simulink model "multilevelinverter1"  (R2014a)
settings: Solver=ode23tb  StartTime=0.0  StopTime=1  RelTol=1e-3
undefined symbols (not defined in the file): a, Gn, Ipvn, Iscn, k, Ki, Kv, Npp, Ns, Nss, q, Rp, Rs, Tn, Vocn
libraries: powerlib x102, simulink x34, dsparch4 x12, powerlib_extras x12, powerlib_meascontrol x3
(part 2 of 2)

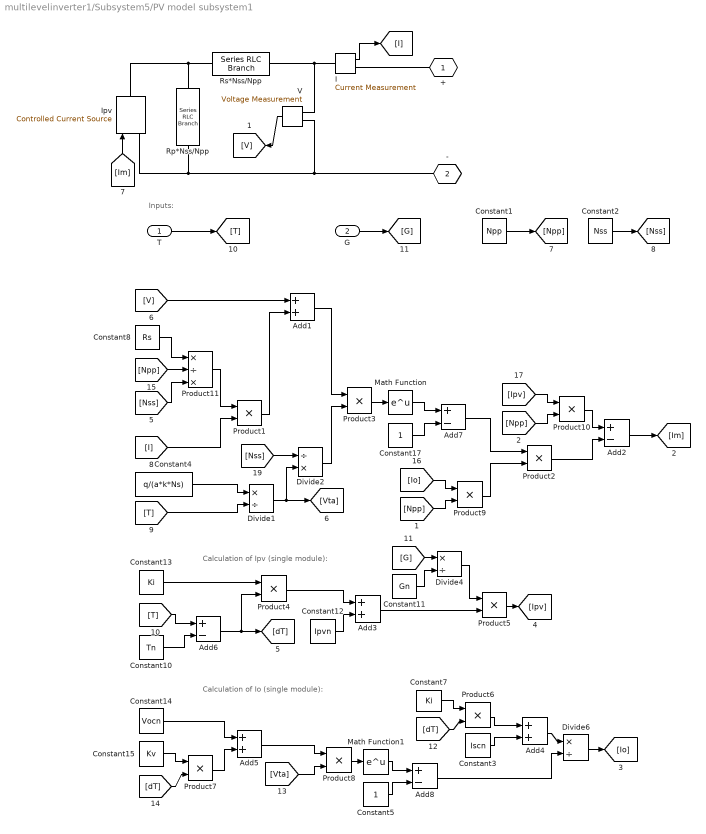
== system multilevelinverter1/Subsystem5/PV model subsystem1 ==
  note: Inputs:
  note: Calculation of Ipv (single module):
  note: Calculation of Io (single module):
  T : Inport
  G : Inport  Port=2
  Add{1,3..5} (4 alike) : Sum
  Add{2,6..8} (4 alike) : Sum  Inputs=+-
  Constant1 : Constant  Value=Npp
  Constant10 : Constant  Value=Tn
  Constant11 : Constant  Value=Gn
  Constant12 : Constant  Value=Ipvn
  Constant13 : Constant  Value=Ki
  Constant14 : Constant  Value=Vocn
  Constant15 : Constant  Value=Kv
  Constant17 : Constant
  Constant2 : Constant  Value=Nss
  Constant3 : Constant  Value=Iscn
  Constant4 : Constant  Value=q/(a*k*Ns)
  Constant5 : Constant
  Constant7 : Constant  Value=Ki
  Constant8 : Constant  Value=Rs
  Divide1 : Product  Inputs=*/
  Divide2 : Product  Inputs=/*
  Divide4 : Product  Inputs=*/
  Divide6 : Product  Inputs=*/
  I : powerlib/Measurements/Current Measurement  PhasorSimulation=off  OutputType=Complex  PSBequivalent=0
  Ipv : powerlib/Electrical Sources/Controlled Current Source  Initialize=on  Source_Type=DC  Amplitude=00  Phase=0  Frequency=0  Measurements=None
  Math Function : Math  SaturateOnIntegerOverflow=on
  Math Function1 : Math  SaturateOnIntegerOverflow=on
  Product{1..10} (10 alike) : Product  RndMeth=Zero
  Product11 : Product  Inputs=*/*  RndMeth=Zero
  Rp*Nss/Npp : powerlib/Elements/Series RLC Branch  LConnTagsString=__new0  RConnTagsString=__new0  BranchType=R  Resistance=Rp*Nss/Npp  Inductance=1e-3  SetiL0=off  InitialCurrent=0  Capacitance=1e-6  Setx0=off  InitialVoltage=0  Measurements=None
  Rs*Nss/Npp : powerlib/Elements/Series RLC Branch  LConnTagsString=__new0  RConnTagsString=__new0  BranchType=R  Resistance=Rs*Nss/Npp  Inductance=1e-3  SetiL0=off  InitialCurrent=0  Capacitance=1e-6  Setx0=off  InitialVoltage=0  Measurements=None
  "V " : powerlib/Measurements/Voltage Measurement  PhasorSimulation=off  OutputType=Complex  PSBequivalent=0
  + : PMIOPort  Port=1  Side=Right
  - : PMIOPort  Port=2  Side=Right
  wires:
  I/1 -> [I]
  "V "/1 -> [V]
  [Im] -> Ipv/1
  G/1 -> [G]
  T/1 -> [T]
  Constant10/1 -> Add6/2
  [T] -> Add6/1
  [I] -> Product1/2
  Constant4/1 -> Divide1/1
  [T] -> Divide1/2
  [V] -> Add1/1
  Product3/1 -> Math Function/1
  Add2/1 -> [Im]
  Add1/1 -> Product3/1
  [G] -> Divide4/1
  Constant11/1 -> Divide4/2
  Constant13/1 -> Product4/1
  [dT] -> Product6/2
  Constant7/1 -> Product6/1
  [dT] -> Product7/2
  Constant14/1 -> Add5/1
  Product8/1 -> Math Function1/1
  Add5/1 -> Product8/1
  Constant17/1 -> Add7/2
  Add7/1 -> Product2/1
  Constant5/1 -> Add8/2
  Math Function1/1 -> Add8/1
  Divide6/1 -> [Io]
  Product5/1 -> [Ipv]
  Product1/1 -> Add1/2
  Math Function/1 -> Add7/1
  Product4/1 -> Add3/1
  Add3/1 -> Product5/2
  Divide4/1 -> Product5/1
  Product7/1 -> Add5/2
  Constant15/1 -> Product7/1
  [Vta] -> Product8/2
  Add8/1 -> Divide6/2
  Constant3/1 -> Add4/2
  Product6/1 -> Add4/1
  Constant12/1 -> Add3/2
  Product2/1 -> Add2/2
  Product9/1 -> Product2/2
  [Io] -> Product9/1
  [Npp] -> Product9/2
  Constant1/1 -> [Npp]
  Constant2/1 -> [Nss]
  [Ipv] -> Product10/1
  [Npp] -> Product10/2
  Product10/1 -> Add2/1
  Constant8/1 -> Product11/1
  [Npp] -> Product11/2
  [Nss] -> Product11/3
  Product11/1 -> Product1/1
  [Nss] -> Divide2/1
  Divide1/1 -> Divide2/2, [Vta]
  Divide2/1 -> Product3/2
  Add6/1 -> [dT], Product4/2
  Add4/1 -> Divide6/1
  connections:
  I/LConn1 -- "V "/LConn1 -- Rs*Nss/Npp/RConn1
  -/RConn1 -- Rp*Nss/Npp/RConn1 -- Ipv/LConn1 -- "V "/LConn2
  Ipv/RConn1 -- Rs*Nss/Npp/LConn1 -- Rp*Nss/Npp/LConn1
  +/RConn1 -- I/RConn1

== system multilevelinverter1/Subsystem6/PV Boost Converter1 ==
  Analog Filter Design : dsparch4/Analog Filter Design  method=Butterworth  filttype=Lowpass  N=8  Wlo=30  Whi=80  Rp=2  Rs=40
  Analog Filter Design1 : dsparch4/Analog Filter Design  method=Butterworth  filttype=Lowpass  N=8  Wlo=30  Whi=80  Rp=2  Rs=40
  Current Measurement : powerlib/Measurements/Current Measurement  PhasorSimulation=off  OutputType=Complex  PSBequivalent=0
  Diode : powerlib/Power Electronics/Diode  Ron=0.001  Lon=0  Vf=0.8  IC=0  UseSnubber=off  Rs=500  Cs=250e-9  Measurements=on
  MPPT : Subsystem
  Mosfet : powerlib/Power Electronics/Mosfet  Ron=0.1  Lon=0  Rd=0.01  Vfd=0  IC=0  Rs=1e5  Cs=inf  Measurements=on
  PI CONTOLER : Subsystem
  Relational Operator1 : RelationalOperator  Operator=<=  OutDataTypeStr=boolean
  Repeating Sequence : simulink/Sources/Repeating Sequence  rep_seq_t=[0 0.0001 0.0002]  rep_seq_y=[0 10 0]
  Scope{1..3,8} (4 alike) : Scope
      Scope1 settings: SaveName=ScopeData2
      Scope2 settings: SaveName=ScopeData3
      Scope3 settings: YMin=-20  YMax=100  SaveName=ScopeData12
      Scope8 settings: YMin=47.1  YMax=48.9  SaveName=ScopeData4
  Series RLC Branch : powerlib/Elements/Series RLC Branch  LConnTagsString=__new0  RConnTagsString=__new0  BranchType=L  Resistance=1  Inductance=1e-3  SetiL0=off  InitialCurrent=0  Capacitance=1e-6  Setx0=off  InitialVoltage=0  Measurements=None
  Series RLC Branch1 : powerlib/Elements/Series RLC Branch  LConnTagsString=__new0  RConnTagsString=__new0  BranchType=C  Resistance=1  Inductance=12e-3  SetiL0=off  InitialCurrent=0  Capacitance=2200e-6  Setx0=off  InitialVoltage=0  Measurements=None
  Voltage Measurement1 : powerlib/Measurements/Voltage Measurement  PhasorSimulation=off  OutputType=Complex  PSBequivalent=0
  Voltage Measurement2 : powerlib/Measurements/Voltage Measurement  PhasorSimulation=off  OutputType=Complex  PSBequivalent=0
  + : PMIOPort  Port=1  Side=Right
  - : PMIOPort  Port=2  Side=Right
  Vpv+ : PMIOPort  Tag=PMCPort  Port=3  Side=Left
  Vpv- : PMIOPort  Tag=PMCPort  Port=4  Side=Left
  wires:
  Analog Filter Design1/1 -> MPPT/1(V)
  Analog Filter Design/1 -> MPPT/2(I)
  MPPT/1(D) -> Relational Operator1/2
  Relational Operator1/1 -> Scope1/1
  Repeating Sequence/1 -> Scope2/1, Relational Operator1/1
  Current Measurement/1 -> Analog Filter Design/1
  Voltage Measurement1/1 -> Scope8/1, [A1]
  [A1] -> PI CONTOLER/1(In1)
  PI CONTOLER/1(Out1) -> [G]
  Voltage Measurement2/1 -> Scope3/1, Analog Filter Design1/1
  [G] -> Mosfet/1
  connections:
  Current Measurement/LConn1 -- Vpv+/RConn1
  Diode/RConn1 -- Voltage Measurement1/LConn1 -- +/RConn1 -- Series RLC Branch1/LConn1
  Series RLC Branch/LConn1 -- Current Measurement/RConn1 -- Voltage Measurement2/LConn1
  Series RLC Branch1/RConn1 -- Voltage Measurement1/LConn2 -- -/RConn1 -- Mosfet/RConn1 -- Voltage Measurement2/LConn2 -- Vpv-/RConn1
  Diode/LConn1 -- Mosfet/LConn1 -- Series RLC Branch/RConn1

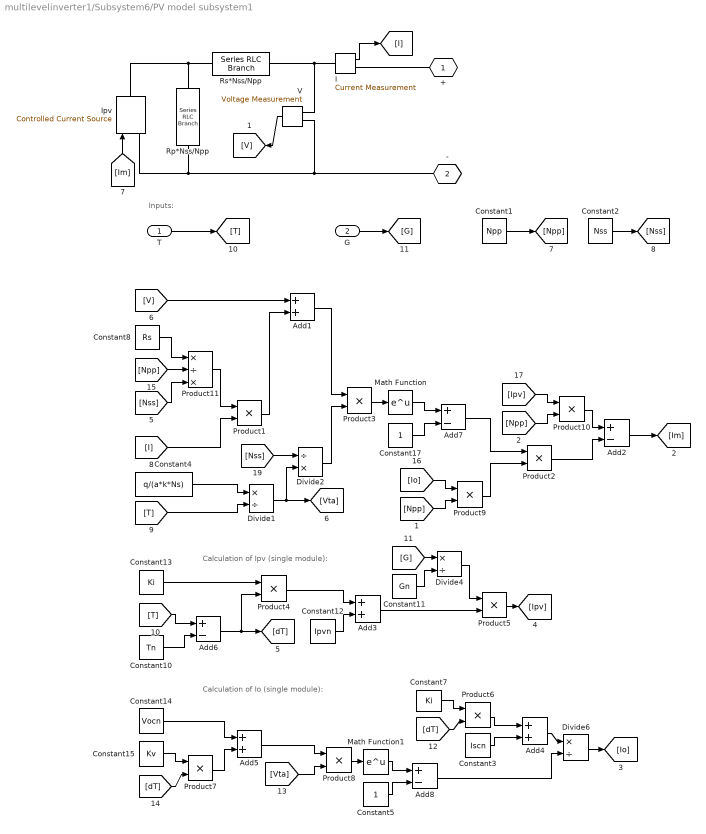
== system multilevelinverter1/Subsystem6/PV model subsystem1 ==
  note: Inputs:
  note: Calculation of Ipv (single module):
  note: Calculation of Io (single module):
  T : Inport
  G : Inport  Port=2
  Add{1,3..5} (4 alike) : Sum
  Add{2,6..8} (4 alike) : Sum  Inputs=+-
  Constant1 : Constant  Value=Npp
  Constant10 : Constant  Value=Tn
  Constant11 : Constant  Value=Gn
  Constant12 : Constant  Value=Ipvn
  Constant13 : Constant  Value=Ki
  Constant14 : Constant  Value=Vocn
  Constant15 : Constant  Value=Kv
  Constant17 : Constant
  Constant2 : Constant  Value=Nss
  Constant3 : Constant  Value=Iscn
  Constant4 : Constant  Value=q/(a*k*Ns)
  Constant5 : Constant
  Constant7 : Constant  Value=Ki
  Constant8 : Constant  Value=Rs
  Divide1 : Product  Inputs=*/
  Divide2 : Product  Inputs=/*
  Divide4 : Product  Inputs=*/
  Divide6 : Product  Inputs=*/
  I : powerlib/Measurements/Current Measurement  PhasorSimulation=off  OutputType=Complex  PSBequivalent=0
  Ipv : powerlib/Electrical Sources/Controlled Current Source  Initialize=on  Source_Type=DC  Amplitude=00  Phase=0  Frequency=0  Measurements=None
  Math Function : Math  SaturateOnIntegerOverflow=on
  Math Function1 : Math  SaturateOnIntegerOverflow=on
  Product{1..10} (10 alike) : Product  RndMeth=Zero
  Product11 : Product  Inputs=*/*  RndMeth=Zero
  Rp*Nss/Npp : powerlib/Elements/Series RLC Branch  LConnTagsString=__new0  RConnTagsString=__new0  BranchType=R  Resistance=Rp*Nss/Npp  Inductance=1e-3  SetiL0=off  InitialCurrent=0  Capacitance=1e-6  Setx0=off  InitialVoltage=0  Measurements=None
  Rs*Nss/Npp : powerlib/Elements/Series RLC Branch  LConnTagsString=__new0  RConnTagsString=__new0  BranchType=R  Resistance=Rs*Nss/Npp  Inductance=1e-3  SetiL0=off  InitialCurrent=0  Capacitance=1e-6  Setx0=off  InitialVoltage=0  Measurements=None
  "V " : powerlib/Measurements/Voltage Measurement  PhasorSimulation=off  OutputType=Complex  PSBequivalent=0
  + : PMIOPort  Port=1  Side=Right
  - : PMIOPort  Port=2  Side=Right
  wires:
  I/1 -> [I]
  "V "/1 -> [V]
  [Im] -> Ipv/1
  G/1 -> [G]
  T/1 -> [T]
  Constant10/1 -> Add6/2
  [T] -> Add6/1
  [I] -> Product1/2
  Constant4/1 -> Divide1/1
  [T] -> Divide1/2
  [V] -> Add1/1
  Product3/1 -> Math Function/1
  Add2/1 -> [Im]
  Add1/1 -> Product3/1
  [G] -> Divide4/1
  Constant11/1 -> Divide4/2
  Constant13/1 -> Product4/1
  [dT] -> Product6/2
  Constant7/1 -> Product6/1
  [dT] -> Product7/2
  Constant14/1 -> Add5/1
  Product8/1 -> Math Function1/1
  Add5/1 -> Product8/1
  Constant17/1 -> Add7/2
  Add7/1 -> Product2/1
  Constant5/1 -> Add8/2
  Math Function1/1 -> Add8/1
  Divide6/1 -> [Io]
  Product5/1 -> [Ipv]
  Product1/1 -> Add1/2
  Math Function/1 -> Add7/1
  Product4/1 -> Add3/1
  Add3/1 -> Product5/2
  Divide4/1 -> Product5/1
  Product7/1 -> Add5/2
  Constant15/1 -> Product7/1
  [Vta] -> Product8/2
  Add8/1 -> Divide6/2
  Constant3/1 -> Add4/2
  Product6/1 -> Add4/1
  Constant12/1 -> Add3/2
  Product2/1 -> Add2/2
  Product9/1 -> Product2/2
  [Io] -> Product9/1
  [Npp] -> Product9/2
  Constant1/1 -> [Npp]
  Constant2/1 -> [Nss]
  [Ipv] -> Product10/1
  [Npp] -> Product10/2
  Product10/1 -> Add2/1
  Constant8/1 -> Product11/1
  [Npp] -> Product11/2
  [Nss] -> Product11/3
  Product11/1 -> Product1/1
  [Nss] -> Divide2/1
  Divide1/1 -> Divide2/2, [Vta]
  Divide2/1 -> Product3/2
  Add6/1 -> [dT], Product4/2
  Add4/1 -> Divide6/1
  connections:
  I/LConn1 -- "V "/LConn1 -- Rs*Nss/Npp/RConn1
  -/RConn1 -- Rp*Nss/Npp/RConn1 -- Ipv/LConn1 -- "V "/LConn2
  Ipv/RConn1 -- Rs*Nss/Npp/LConn1 -- Rp*Nss/Npp/LConn1
  +/RConn1 -- I/RConn1

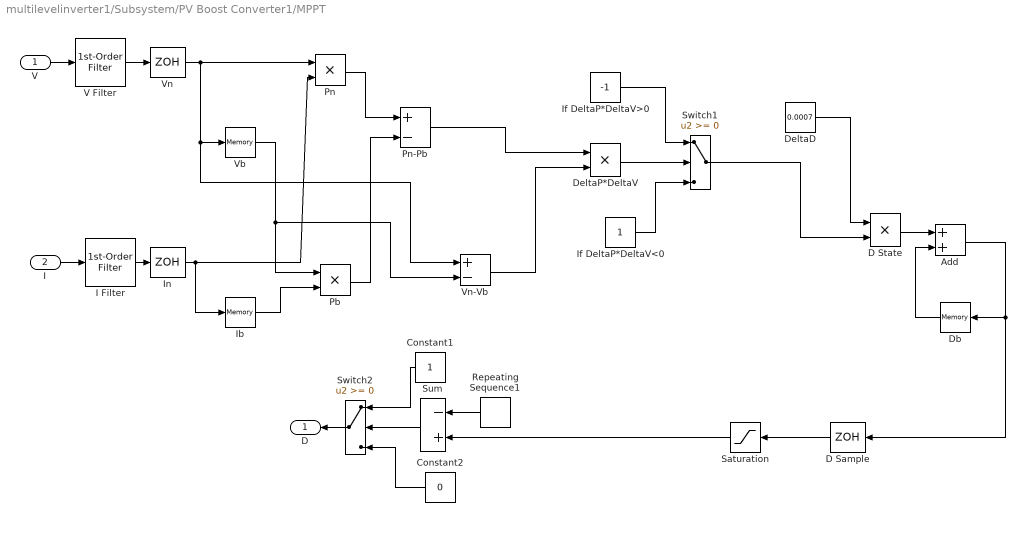
== system multilevelinverter1/Subsystem/PV Boost Converter1/MPPT ==
  V : Inport
  I : Inport  Port=2
  Add : Sum
  Constant1 : Constant  SampleTime=-1
  Constant2 : Constant  Value=0  SampleTime=-1
  D Sample : ZeroOrderHold  SampleTime=1e-4
  D State : Product  RndMeth=Zero
  Db : Memory  InheritSampleTime=on
  DeltaD : Constant  Value=0.0007
  DeltaP*DeltaV : Product  RndMeth=Zero
  I Filter : powerlib_extras/Control  Blocks/1st-Order  Filter  FilterType=Lowpass  Tc=1e-3  Initialize=off  Vac_Init=[0.8 -25 60]  Vdc_Init=-0.4  PlotResponse=off  param1=[1 500 1]
  Ib : Memory  InheritSampleTime=on
  If DeltaP*DeltaV<0 : Constant
  If DeltaP*DeltaV>0 : Constant  Value=-1
  In : ZeroOrderHold  SampleTime=1e-4
  Pb : Product  RndMeth=Zero
  Pn : Product  RndMeth=Zero
  Pn-Pb : Sum  Inputs=+-
  Repeating Sequence1 : simulink/Sources/Repeating Sequence  rep_seq_t=[0 4e-3 8e-3]  rep_seq_y=[0 1 0]
  Saturation : Saturate  UpperLimit=0.8  LowerLimit=0
  Sum : Sum  Inputs=-+  SaturateOnIntegerOverflow=on
  Switch1 : Switch
  Switch2 : Switch
  V Filter : powerlib_extras/Control  Blocks/1st-Order  Filter  FilterType=Lowpass  Tc=1e-3  Initialize=off  Vac_Init=[0.8 -25 60]  Vdc_Init=-0.4  PlotResponse=off  param1=[1 500 1]
  Vb : Memory  InheritSampleTime=on
  Vn : ZeroOrderHold  SampleTime=1e-4
  Vn-Vb : Sum  Inputs=+-
  D : Outport
  wires:
  Saturation/1 -> Sum/2
  DeltaD/1 -> D State/1
  Switch1/1 -> D State/2
  If DeltaP*DeltaV<0/1 -> Switch1/3
  If DeltaP*DeltaV>0/1 -> Switch1/1
  DeltaP*DeltaV/1 -> Switch1/2
  Vn-Vb/1 -> DeltaP*DeltaV/2
  Pn-Pb/1 -> DeltaP*DeltaV/1
  D Sample/1 -> Saturation/1
  Db/1 -> Add/2
  Switch2/1 -> D/1
  Add/1 -> D Sample/1, Db/1
  Repeating Sequence1/1 -> Sum/1
  Sum/1 -> Switch2/2
  Constant1/1 -> Switch2/1
  Constant2/1 -> Switch2/3
  D State/1 -> Add/1
  Pb/1 -> Pn-Pb/2
  Pn/1 -> Pn-Pb/1
  Vb/1 -> Vn-Vb/2, Pb/1
  Ib/1 -> Pb/2
  Vn/1 -> Vn-Vb/1, Vb/1, Pn/1
  In/1 -> Pn/2, Ib/1
  I Filter/1 -> In/1
  V Filter/1 -> Vn/1
  I/1 -> I Filter/1
  V/1 -> V Filter/1

== system multilevelinverter1/Subsystem/PV Boost Converter1/PI CONTOLER ==
  In1 : Inport
  Add : Sum  Inputs=+-
  Constant1 : Constant  Value=48
  Gain1 : Gain  Gain=0.1
  Gain2 : Gain  Gain=10
  Integrator : Integrator
  Mux : Mux  Inputs=2
  Ramp1 : simulink/Sources/Ramp  slope=1  start=0  X0=0
  Relational Operator1 : RelationalOperator  OutDataTypeStr=boolean
  Repeating Sequence : simulink/Sources/Repeating Sequence  rep_seq_t=[0 0.0001 0.0002]  rep_seq_y=[0 10 0]
  Saturation1 : Saturate  UpperLimit=10  LowerLimit=0
  Scope{1..5} (5 alike) : Scope
      Scope1 settings: SaveName=ScopeData6
      Scope2 settings: SaveName=ScopeData7
      Scope3 settings: SaveName=ScopeData8
      Scope4 settings: SaveName=ScopeData9
      Scope5 settings: SaveName=ScopeData10
  Sum : Sum  Inputs=|++
  Out1 : Outport
  wires:
  Saturation1/1 -> Relational Operator1/2, Scope5/1
  Gain2/1 -> Integrator/1
  In1/1 -> Mux/2, Add/2
  Sum/1 -> Saturation1/1, Scope2/1
  Mux/1 -> Scope4/1
  Integrator/1 -> Sum/2
  Gain1/1 -> Sum/1
  Relational Operator1/1 -> Out1/1, Scope1/1
  Repeating Sequence/1 -> Scope3/1, Relational Operator1/1
  Add/1 -> Gain2/1, Gain1/1
  Constant1/1 -> Mux/1, Add/1

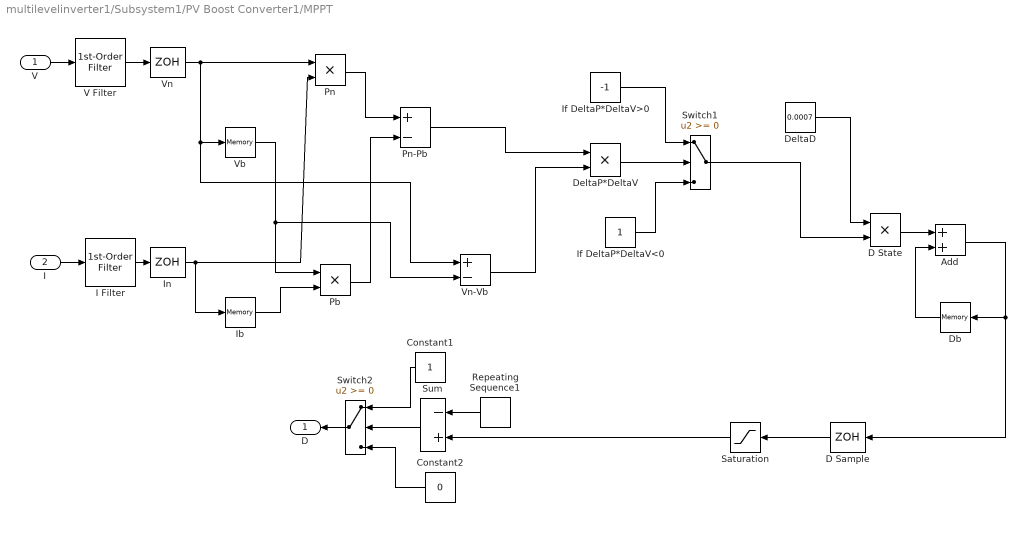
== system multilevelinverter1/Subsystem1/PV Boost Converter1/MPPT ==
  V : Inport
  I : Inport  Port=2
  Add : Sum
  Constant1 : Constant  SampleTime=-1
  Constant2 : Constant  Value=0  SampleTime=-1
  D Sample : ZeroOrderHold  SampleTime=1e-4
  D State : Product  RndMeth=Zero
  Db : Memory  InheritSampleTime=on
  DeltaD : Constant  Value=0.0007
  DeltaP*DeltaV : Product  RndMeth=Zero
  I Filter : powerlib_extras/Control  Blocks/1st-Order  Filter  FilterType=Lowpass  Tc=1e-3  Initialize=off  Vac_Init=[0.8 -25 60]  Vdc_Init=-0.4  PlotResponse=off  param1=[1 500 1]
  Ib : Memory  InheritSampleTime=on
  If DeltaP*DeltaV<0 : Constant
  If DeltaP*DeltaV>0 : Constant  Value=-1
  In : ZeroOrderHold  SampleTime=1e-4
  Pb : Product  RndMeth=Zero
  Pn : Product  RndMeth=Zero
  Pn-Pb : Sum  Inputs=+-
  Repeating Sequence1 : simulink/Sources/Repeating Sequence  rep_seq_t=[0 4e-3 8e-3]  rep_seq_y=[0 1 0]
  Saturation : Saturate  UpperLimit=0.8  LowerLimit=0
  Sum : Sum  Inputs=-+  SaturateOnIntegerOverflow=on
  Switch1 : Switch
  Switch2 : Switch
  V Filter : powerlib_extras/Control  Blocks/1st-Order  Filter  FilterType=Lowpass  Tc=1e-3  Initialize=off  Vac_Init=[0.8 -25 60]  Vdc_Init=-0.4  PlotResponse=off  param1=[1 500 1]
  Vb : Memory  InheritSampleTime=on
  Vn : ZeroOrderHold  SampleTime=1e-4
  Vn-Vb : Sum  Inputs=+-
  D : Outport
  wires:
  V/1 -> V Filter/1
  I/1 -> I Filter/1
  V Filter/1 -> Vn/1
  I Filter/1 -> In/1
  In/1 -> Ib/1, Pn/2
  Vn/1 -> Pn/1, Vb/1, Vn-Vb/1
  Ib/1 -> Pb/2
  Vb/1 -> Pb/1, Vn-Vb/2
  Pn/1 -> Pn-Pb/1
  Pb/1 -> Pn-Pb/2
  D State/1 -> Add/1
  Constant2/1 -> Switch2/3
  Constant1/1 -> Switch2/1
  Sum/1 -> Switch2/2
  Repeating Sequence1/1 -> Sum/1
  Add/1 -> Db/1, D Sample/1
  Switch2/1 -> D/1
  Db/1 -> Add/2
  D Sample/1 -> Saturation/1
  Pn-Pb/1 -> DeltaP*DeltaV/1
  Vn-Vb/1 -> DeltaP*DeltaV/2
  DeltaP*DeltaV/1 -> Switch1/2
  If DeltaP*DeltaV>0/1 -> Switch1/1
  If DeltaP*DeltaV<0/1 -> Switch1/3
  Switch1/1 -> D State/2
  DeltaD/1 -> D State/1
  Saturation/1 -> Sum/2

== system multilevelinverter1/Subsystem1/PV Boost Converter1/PI CONTOLER ==
  In1 : Inport
  Add : Sum  Inputs=+-
  Constant1 : Constant  Value=48
  Gain1 : Gain  Gain=0.1
  Gain2 : Gain  Gain=10
  Integrator : Integrator
  Mux : Mux  Inputs=2
  Ramp1 : simulink/Sources/Ramp  slope=1  start=0  X0=0
  Relational Operator1 : RelationalOperator  OutDataTypeStr=boolean
  Repeating Sequence : simulink/Sources/Repeating Sequence  rep_seq_t=[0 0.0001 0.0002]  rep_seq_y=[0 10 0]
  Saturation1 : Saturate  UpperLimit=10  LowerLimit=0
  Scope{1..5} (5 alike) : Scope
      Scope1 settings: SaveName=ScopeData6
      Scope2 settings: SaveName=ScopeData7
      Scope3 settings: SaveName=ScopeData8
      Scope4 settings: SaveName=ScopeData9
      Scope5 settings: SaveName=ScopeData10
  Sum : Sum  Inputs=|++
  Out1 : Outport
  wires:
  Constant1/1 -> Add/1, Mux/1
  Add/1 -> Gain1/1, Gain2/1
  Repeating Sequence/1 -> Relational Operator1/1, Scope3/1
  Relational Operator1/1 -> Scope1/1, Out1/1
  Gain1/1 -> Sum/1
  Integrator/1 -> Sum/2
  Mux/1 -> Scope4/1
  Sum/1 -> Scope2/1, Saturation1/1
  In1/1 -> Add/2, Mux/2
  Gain2/1 -> Integrator/1
  Saturation1/1 -> Scope5/1, Relational Operator1/2

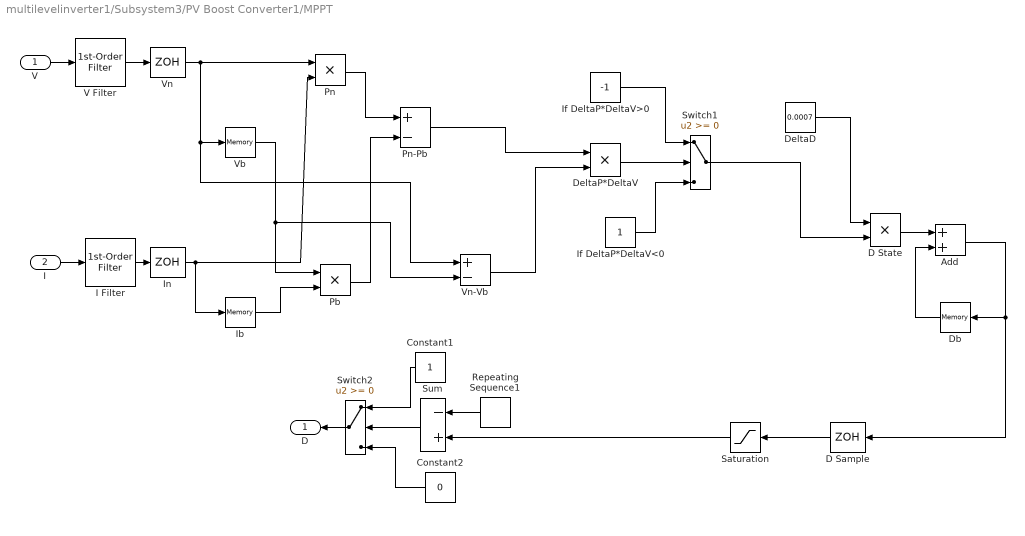
== system multilevelinverter1/Subsystem3/PV Boost Converter1/MPPT ==
  V : Inport
  I : Inport  Port=2
  Add : Sum
  Constant1 : Constant  SampleTime=-1
  Constant2 : Constant  Value=0  SampleTime=-1
  D Sample : ZeroOrderHold  SampleTime=1e-4
  D State : Product  RndMeth=Zero
  Db : Memory  InheritSampleTime=on
  DeltaD : Constant  Value=0.0007
  DeltaP*DeltaV : Product  RndMeth=Zero
  I Filter : powerlib_extras/Control  Blocks/1st-Order  Filter  FilterType=Lowpass  Tc=1e-3  Initialize=off  Vac_Init=[0.8 -25 60]  Vdc_Init=-0.4  PlotResponse=off  param1=[1 500 1]
  Ib : Memory  InheritSampleTime=on
  If DeltaP*DeltaV<0 : Constant
  If DeltaP*DeltaV>0 : Constant  Value=-1
  In : ZeroOrderHold  SampleTime=1e-4
  Pb : Product  RndMeth=Zero
  Pn : Product  RndMeth=Zero
  Pn-Pb : Sum  Inputs=+-
  Repeating Sequence1 : simulink/Sources/Repeating Sequence  rep_seq_t=[0 4e-3 8e-3]  rep_seq_y=[0 1 0]
  Saturation : Saturate  UpperLimit=0.8  LowerLimit=0
  Sum : Sum  Inputs=-+  SaturateOnIntegerOverflow=on
  Switch1 : Switch
  Switch2 : Switch
  V Filter : powerlib_extras/Control  Blocks/1st-Order  Filter  FilterType=Lowpass  Tc=1e-3  Initialize=off  Vac_Init=[0.8 -25 60]  Vdc_Init=-0.4  PlotResponse=off  param1=[1 500 1]
  Vb : Memory  InheritSampleTime=on
  Vn : ZeroOrderHold  SampleTime=1e-4
  Vn-Vb : Sum  Inputs=+-
  D : Outport
  wires:
  V/1 -> V Filter/1
  I/1 -> I Filter/1
  V Filter/1 -> Vn/1
  I Filter/1 -> In/1
  In/1 -> Ib/1, Pn/2
  Vn/1 -> Pn/1, Vb/1, Vn-Vb/1
  Ib/1 -> Pb/2
  Vb/1 -> Pb/1, Vn-Vb/2
  Pn/1 -> Pn-Pb/1
  Pb/1 -> Pn-Pb/2
  D State/1 -> Add/1
  Constant2/1 -> Switch2/3
  Constant1/1 -> Switch2/1
  Sum/1 -> Switch2/2
  Repeating Sequence1/1 -> Sum/1
  Add/1 -> Db/1, D Sample/1
  Switch2/1 -> D/1
  Db/1 -> Add/2
  D Sample/1 -> Saturation/1
  Pn-Pb/1 -> DeltaP*DeltaV/1
  Vn-Vb/1 -> DeltaP*DeltaV/2
  DeltaP*DeltaV/1 -> Switch1/2
  If DeltaP*DeltaV>0/1 -> Switch1/1
  If DeltaP*DeltaV<0/1 -> Switch1/3
  Switch1/1 -> D State/2
  DeltaD/1 -> D State/1
  Saturation/1 -> Sum/2

== system multilevelinverter1/Subsystem3/PV Boost Converter1/PI CONTOLER ==
  In1 : Inport
  Add : Sum  Inputs=+-
  Constant1 : Constant  Value=48
  Gain1 : Gain  Gain=0.1
  Gain2 : Gain  Gain=10
  Integrator : Integrator
  Mux : Mux  Inputs=2
  Ramp1 : simulink/Sources/Ramp  slope=1  start=0  X0=0
  Relational Operator1 : RelationalOperator  OutDataTypeStr=boolean
  Repeating Sequence : simulink/Sources/Repeating Sequence  rep_seq_t=[0 0.0001 0.0002]  rep_seq_y=[0 10 0]
  Saturation1 : Saturate  UpperLimit=10  LowerLimit=0
  Scope{1..5} (5 alike) : Scope
      Scope1 settings: SaveName=ScopeData6
      Scope2 settings: SaveName=ScopeData7
      Scope3 settings: SaveName=ScopeData8
      Scope4 settings: SaveName=ScopeData9
      Scope5 settings: SaveName=ScopeData10
  Sum : Sum  Inputs=|++
  Out1 : Outport
  wires:
  Constant1/1 -> Add/1, Mux/1
  Add/1 -> Gain1/1, Gain2/1
  Repeating Sequence/1 -> Relational Operator1/1, Scope3/1
  Relational Operator1/1 -> Scope1/1, Out1/1
  Gain1/1 -> Sum/1
  Integrator/1 -> Sum/2
  Mux/1 -> Scope4/1
  Sum/1 -> Scope2/1, Saturation1/1
  In1/1 -> Add/2, Mux/2
  Gain2/1 -> Integrator/1
  Saturation1/1 -> Scope5/1, Relational Operator1/2

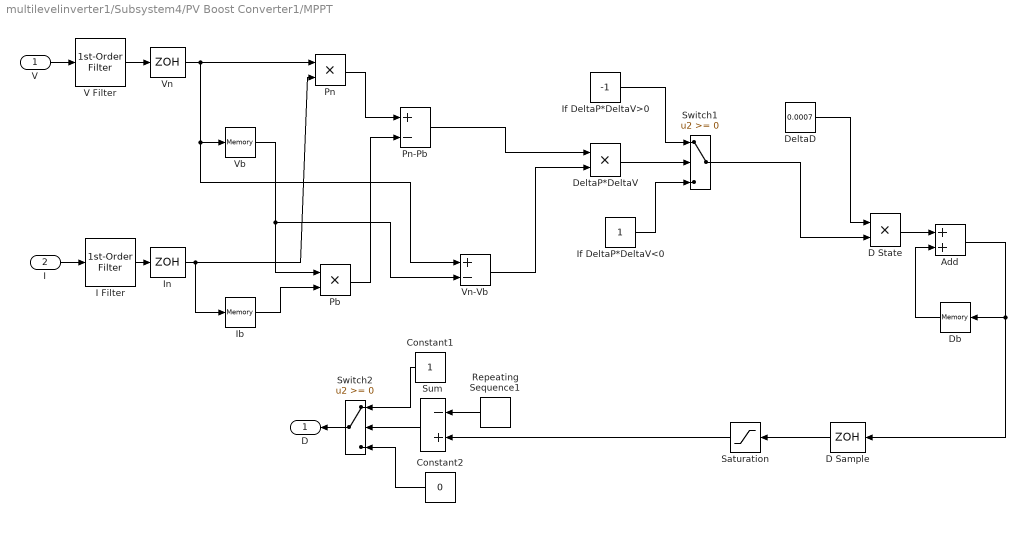
== system multilevelinverter1/Subsystem4/PV Boost Converter1/MPPT ==
  V : Inport
  I : Inport  Port=2
  Add : Sum
  Constant1 : Constant  SampleTime=-1
  Constant2 : Constant  Value=0  SampleTime=-1
  D Sample : ZeroOrderHold  SampleTime=1e-4
  D State : Product  RndMeth=Zero
  Db : Memory  InheritSampleTime=on
  DeltaD : Constant  Value=0.0007
  DeltaP*DeltaV : Product  RndMeth=Zero
  I Filter : powerlib_extras/Control  Blocks/1st-Order  Filter  FilterType=Lowpass  Tc=1e-3  Initialize=off  Vac_Init=[0.8 -25 60]  Vdc_Init=-0.4  PlotResponse=off  param1=[1 500 1]
  Ib : Memory  InheritSampleTime=on
  If DeltaP*DeltaV<0 : Constant
  If DeltaP*DeltaV>0 : Constant  Value=-1
  In : ZeroOrderHold  SampleTime=1e-4
  Pb : Product  RndMeth=Zero
  Pn : Product  RndMeth=Zero
  Pn-Pb : Sum  Inputs=+-
  Repeating Sequence1 : simulink/Sources/Repeating Sequence  rep_seq_t=[0 4e-3 8e-3]  rep_seq_y=[0 1 0]
  Saturation : Saturate  UpperLimit=0.8  LowerLimit=0
  Sum : Sum  Inputs=-+  SaturateOnIntegerOverflow=on
  Switch1 : Switch
  Switch2 : Switch
  V Filter : powerlib_extras/Control  Blocks/1st-Order  Filter  FilterType=Lowpass  Tc=1e-3  Initialize=off  Vac_Init=[0.8 -25 60]  Vdc_Init=-0.4  PlotResponse=off  param1=[1 500 1]
  Vb : Memory  InheritSampleTime=on
  Vn : ZeroOrderHold  SampleTime=1e-4
  Vn-Vb : Sum  Inputs=+-
  D : Outport
  wires:
  V/1 -> V Filter/1
  I/1 -> I Filter/1
  V Filter/1 -> Vn/1
  I Filter/1 -> In/1
  In/1 -> Ib/1, Pn/2
  Vn/1 -> Pn/1, Vb/1, Vn-Vb/1
  Ib/1 -> Pb/2
  Vb/1 -> Pb/1, Vn-Vb/2
  Pn/1 -> Pn-Pb/1
  Pb/1 -> Pn-Pb/2
  D State/1 -> Add/1
  Constant2/1 -> Switch2/3
  Constant1/1 -> Switch2/1
  Sum/1 -> Switch2/2
  Repeating Sequence1/1 -> Sum/1
  Add/1 -> Db/1, D Sample/1
  Switch2/1 -> D/1
  Db/1 -> Add/2
  D Sample/1 -> Saturation/1
  Pn-Pb/1 -> DeltaP*DeltaV/1
  Vn-Vb/1 -> DeltaP*DeltaV/2
  DeltaP*DeltaV/1 -> Switch1/2
  If DeltaP*DeltaV>0/1 -> Switch1/1
  If DeltaP*DeltaV<0/1 -> Switch1/3
  Switch1/1 -> D State/2
  DeltaD/1 -> D State/1
  Saturation/1 -> Sum/2

== system multilevelinverter1/Subsystem4/PV Boost Converter1/PI CONTOLER ==
  In1 : Inport
  Add : Sum  Inputs=+-
  Constant1 : Constant  Value=48
  Gain1 : Gain  Gain=0.1
  Gain2 : Gain  Gain=10
  Integrator : Integrator
  Mux : Mux  Inputs=2
  Ramp1 : simulink/Sources/Ramp  slope=1  start=0  X0=0
  Relational Operator1 : RelationalOperator  OutDataTypeStr=boolean
  Repeating Sequence : simulink/Sources/Repeating Sequence  rep_seq_t=[0 0.0001 0.0002]  rep_seq_y=[0 10 0]
  Saturation1 : Saturate  UpperLimit=10  LowerLimit=0
  Scope{1..5} (5 alike) : Scope
      Scope1 settings: SaveName=ScopeData6
      Scope2 settings: SaveName=ScopeData7
      Scope3 settings: SaveName=ScopeData8
      Scope4 settings: SaveName=ScopeData9
      Scope5 settings: SaveName=ScopeData10
  Sum : Sum  Inputs=|++
  Out1 : Outport
  wires:
  Constant1/1 -> Add/1, Mux/1
  Add/1 -> Gain1/1, Gain2/1
  Repeating Sequence/1 -> Relational Operator1/1, Scope3/1
  Relational Operator1/1 -> Scope1/1, Out1/1
  Gain1/1 -> Sum/1
  Integrator/1 -> Sum/2
  Mux/1 -> Scope4/1
  Sum/1 -> Scope2/1, Saturation1/1
  In1/1 -> Add/2, Mux/2
  Gain2/1 -> Integrator/1
  Saturation1/1 -> Scope5/1, Relational Operator1/2

== system multilevelinverter1/Subsystem5/PV Boost Converter1/MPPT ==
  V : Inport
  I : Inport  Port=2
  Add : Sum
  Constant1 : Constant  SampleTime=-1
  Constant2 : Constant  Value=0  SampleTime=-1
  D Sample : ZeroOrderHold  SampleTime=1e-4
  D State : Product  RndMeth=Zero
  Db : Memory  InheritSampleTime=on
  DeltaD : Constant  Value=0.0007
  DeltaP*DeltaV : Product  RndMeth=Zero
  I Filter : powerlib_extras/Control  Blocks/1st-Order  Filter  FilterType=Lowpass  Tc=1e-3  Initialize=off  Vac_Init=[0.8 -25 60]  Vdc_Init=-0.4  PlotResponse=off  param1=[1 500 1]
  Ib : Memory  InheritSampleTime=on
  If DeltaP*DeltaV<0 : Constant
  If DeltaP*DeltaV>0 : Constant  Value=-1
  In : ZeroOrderHold  SampleTime=1e-4
  Pb : Product  RndMeth=Zero
  Pn : Product  RndMeth=Zero
  Pn-Pb : Sum  Inputs=+-
  Repeating Sequence1 : simulink/Sources/Repeating Sequence  rep_seq_t=[0 4e-3 8e-3]  rep_seq_y=[0 1 0]
  Saturation : Saturate  UpperLimit=0.8  LowerLimit=0
  Sum : Sum  Inputs=-+  SaturateOnIntegerOverflow=on
  Switch1 : Switch
  Switch2 : Switch
  V Filter : powerlib_extras/Control  Blocks/1st-Order  Filter  FilterType=Lowpass  Tc=1e-3  Initialize=off  Vac_Init=[0.8 -25 60]  Vdc_Init=-0.4  PlotResponse=off  param1=[1 500 1]
  Vb : Memory  InheritSampleTime=on
  Vn : ZeroOrderHold  SampleTime=1e-4
  Vn-Vb : Sum  Inputs=+-
  D : Outport
  wires:
  Saturation/1 -> Sum/2
  DeltaD/1 -> D State/1
  Switch1/1 -> D State/2
  If DeltaP*DeltaV<0/1 -> Switch1/3
  If DeltaP*DeltaV>0/1 -> Switch1/1
  DeltaP*DeltaV/1 -> Switch1/2
  Vn-Vb/1 -> DeltaP*DeltaV/2
  Pn-Pb/1 -> DeltaP*DeltaV/1
  D Sample/1 -> Saturation/1
  Db/1 -> Add/2
  Switch2/1 -> D/1
  Add/1 -> D Sample/1, Db/1
  Repeating Sequence1/1 -> Sum/1
  Sum/1 -> Switch2/2
  Constant1/1 -> Switch2/1
  Constant2/1 -> Switch2/3
  D State/1 -> Add/1
  Pb/1 -> Pn-Pb/2
  Pn/1 -> Pn-Pb/1
  Vb/1 -> Vn-Vb/2, Pb/1
  Ib/1 -> Pb/2
  Vn/1 -> Vn-Vb/1, Vb/1, Pn/1
  In/1 -> Pn/2, Ib/1
  I Filter/1 -> In/1
  V Filter/1 -> Vn/1
  I/1 -> I Filter/1
  V/1 -> V Filter/1

== system multilevelinverter1/Subsystem5/PV Boost Converter1/PI CONTOLER ==
  In1 : Inport
  Add : Sum  Inputs=+-
  Constant1 : Constant  Value=48
  Gain1 : Gain  Gain=0.1
  Gain2 : Gain  Gain=10
  Integrator : Integrator
  Mux : Mux  Inputs=2
  Ramp1 : simulink/Sources/Ramp  slope=1  start=0  X0=0
  Relational Operator1 : RelationalOperator  OutDataTypeStr=boolean
  Repeating Sequence : simulink/Sources/Repeating Sequence  rep_seq_t=[0 0.0001 0.0002]  rep_seq_y=[0 10 0]
  Saturation1 : Saturate  UpperLimit=10  LowerLimit=0
  Scope{1..5} (5 alike) : Scope
      Scope1 settings: SaveName=ScopeData6
      Scope2 settings: SaveName=ScopeData7
      Scope3 settings: SaveName=ScopeData8
      Scope4 settings: SaveName=ScopeData9
      Scope5 settings: SaveName=ScopeData10
  Sum : Sum  Inputs=|++
  Out1 : Outport
  wires:
  Saturation1/1 -> Relational Operator1/2, Scope5/1
  Gain2/1 -> Integrator/1
  In1/1 -> Mux/2, Add/2
  Sum/1 -> Saturation1/1, Scope2/1
  Mux/1 -> Scope4/1
  Integrator/1 -> Sum/2
  Gain1/1 -> Sum/1
  Relational Operator1/1 -> Out1/1, Scope1/1
  Repeating Sequence/1 -> Scope3/1, Relational Operator1/1
  Add/1 -> Gain2/1, Gain1/1
  Constant1/1 -> Mux/1, Add/1

== system multilevelinverter1/Subsystem6/PV Boost Converter1/MPPT ==
  V : Inport
  I : Inport  Port=2
  Add : Sum
  Constant1 : Constant  SampleTime=-1
  Constant2 : Constant  Value=0  SampleTime=-1
  D Sample : ZeroOrderHold  SampleTime=1e-4
  D State : Product  RndMeth=Zero
  Db : Memory  InheritSampleTime=on
  DeltaD : Constant  Value=0.0007
  DeltaP*DeltaV : Product  RndMeth=Zero
  I Filter : powerlib_extras/Control  Blocks/1st-Order  Filter  FilterType=Lowpass  Tc=1e-3  Initialize=off  Vac_Init=[0.8 -25 60]  Vdc_Init=-0.4  PlotResponse=off  param1=[1 500 1]
  Ib : Memory  InheritSampleTime=on
  If DeltaP*DeltaV<0 : Constant
  If DeltaP*DeltaV>0 : Constant  Value=-1
  In : ZeroOrderHold  SampleTime=1e-4
  Pb : Product  RndMeth=Zero
  Pn : Product  RndMeth=Zero
  Pn-Pb : Sum  Inputs=+-
  Repeating Sequence1 : simulink/Sources/Repeating Sequence  rep_seq_t=[0 4e-3 8e-3]  rep_seq_y=[0 1 0]
  Saturation : Saturate  UpperLimit=0.8  LowerLimit=0
  Sum : Sum  Inputs=-+  SaturateOnIntegerOverflow=on
  Switch1 : Switch
  Switch2 : Switch
  V Filter : powerlib_extras/Control  Blocks/1st-Order  Filter  FilterType=Lowpass  Tc=1e-3  Initialize=off  Vac_Init=[0.8 -25 60]  Vdc_Init=-0.4  PlotResponse=off  param1=[1 500 1]
  Vb : Memory  InheritSampleTime=on
  Vn : ZeroOrderHold  SampleTime=1e-4
  Vn-Vb : Sum  Inputs=+-
  D : Outport
  wires:
  Saturation/1 -> Sum/2
  DeltaD/1 -> D State/1
  Switch1/1 -> D State/2
  If DeltaP*DeltaV<0/1 -> Switch1/3
  If DeltaP*DeltaV>0/1 -> Switch1/1
  DeltaP*DeltaV/1 -> Switch1/2
  Vn-Vb/1 -> DeltaP*DeltaV/2
  Pn-Pb/1 -> DeltaP*DeltaV/1
  D Sample/1 -> Saturation/1
  Db/1 -> Add/2
  Switch2/1 -> D/1
  Add/1 -> D Sample/1, Db/1
  Repeating Sequence1/1 -> Sum/1
  Sum/1 -> Switch2/2
  Constant1/1 -> Switch2/1
  Constant2/1 -> Switch2/3
  D State/1 -> Add/1
  Pb/1 -> Pn-Pb/2
  Pn/1 -> Pn-Pb/1
  Vb/1 -> Vn-Vb/2, Pb/1
  Ib/1 -> Pb/2
  Vn/1 -> Vn-Vb/1, Vb/1, Pn/1
  In/1 -> Pn/2, Ib/1
  I Filter/1 -> In/1
  V Filter/1 -> Vn/1
  I/1 -> I Filter/1
  V/1 -> V Filter/1

== system multilevelinverter1/Subsystem6/PV Boost Converter1/PI CONTOLER ==
  In1 : Inport
  Add : Sum  Inputs=+-
  Constant1 : Constant  Value=48
  Gain1 : Gain  Gain=0.5
  Gain2 : Gain  Gain=5
  Integrator : Integrator
  Mean : powerlib_meascontrol/Measurements/Mean  Freq=5000  Vinit=0  Ts=0
  Mean (Variable Frequency) : powerlib_meascontrol/Measurements/Mean (Variable Frequency)  Finit=60  Fmin=45  Vinit=0  Ts=0
  Mux : Mux  Inputs=2
  Ramp1 : simulink/Sources/Ramp  slope=1  start=0  X0=0
  Relational Operator1 : RelationalOperator  OutDataTypeStr=boolean
  Repeating Sequence : simulink/Sources/Repeating Sequence  rep_seq_t=[0 0.0001 0.0002]  rep_seq_y=[0 10 0]
  Saturation1 : Saturate  UpperLimit=10  LowerLimit=0
  Scope{1..5} (5 alike) : Scope
      Scope1 settings: SaveName=ScopeData6
      Scope2 settings: SaveName=ScopeData7
      Scope3 settings: SaveName=ScopeData8
      Scope4 settings: SaveName=ScopeData9
      Scope5 settings: SaveName=ScopeData10
  Sum : Sum  Inputs=|++
  Out1 : Outport
  wires:
  Saturation1/1 -> Relational Operator1/2, Scope5/1
  Gain2/1 -> Integrator/1
  In1/1 -> Mean/1
  Sum/1 -> Saturation1/1, Scope2/1
  Mux/1 -> Scope4/1
  Integrator/1 -> Sum/2
  Gain1/1 -> Sum/1
  Relational Operator1/1 -> Out1/1, Scope1/1
  Repeating Sequence/1 -> Scope3/1, Relational Operator1/1
  Add/1 -> Gain2/1, Gain1/1
  Constant1/1 -> Add/1, Mux/1
  Mean/1 -> Mux/2, Add/2
